simulink model "omav_LBF_bisection_combined"  (R2020a)
settings: Solver=VariableStepAuto  StartTime=0.0  StopTime=20  RelTol=1e-3
undefined symbols (not defined in the file): params
libraries: simulink x13, vrlib x2
settings Model: Creator=daniel  LastModifiedBy=daniel

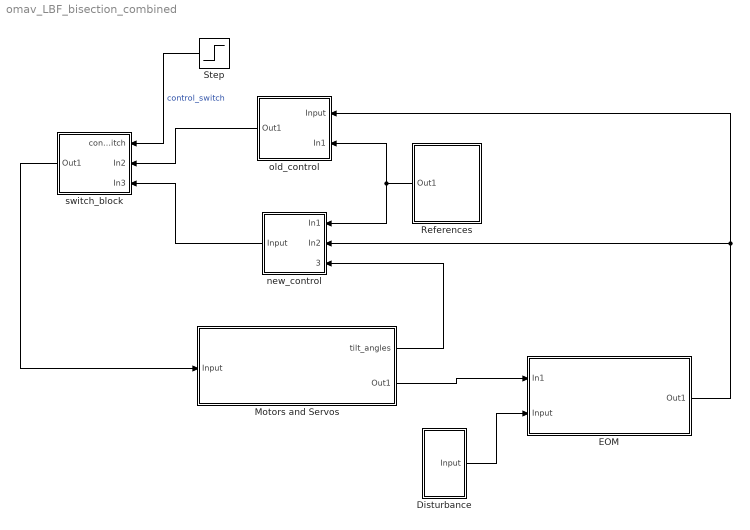
== system omav_LBF_bisection_combined ==
  Disturbance : Subsystem
  EOM : Subsystem
  Motors and Servos : Subsystem
  References : Subsystem
  Step : Step  Time=5  Before=1  After=0  SampleTime=0
  new_control : Subsystem
  old_control : Subsystem
  switch_block : Subsystem
  wires:
  EOM/1(Out1) -> old_control/1(Input), new_control/2(In2)
  References/1(Out1) -> old_control/2(In1), new_control/1(In1)
  Motors and Servos/2(Out1) -> EOM/1(In1)
  Disturbance/1(Input) -> EOM/2(Input)
  Motors and Servos/1(tilt_angles) -> new_control/3(tilt_angles)
  Step/1 -> switch_block/1(control_switch)  "control_switch"
  old_control/1(Out1) -> switch_block/2(In2)
  new_control/1(Input) -> switch_block/3(In3)
  switch_block/1(Out1) -> Motors and Servos/1(Input)

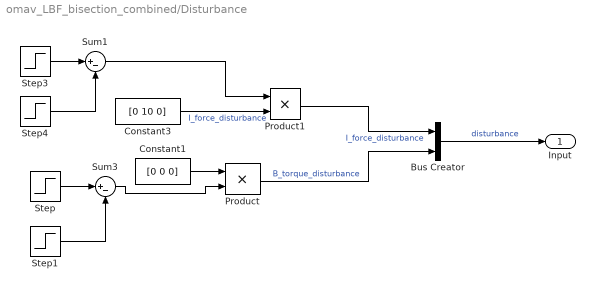
== system omav_LBF_bisection_combined/Disturbance ==
  Bus Creator : BusCreator  Inputs=2
  Constant1 : Constant  Value=[0 0 0]
  Constant3 : Constant  Value=[0 10 0]
  Product : Product
  Product1 : Product
  Step : Step  SampleTime=0
  Step1 : Step  Time=3  SampleTime=0
  Step3 : Step  Time=7  SampleTime=0
  Step4 : Step  Time=8  SampleTime=0
  Sum1 : Sum  Inputs=|+-
  Sum3 : Sum  Inputs=|+-
  Input : Outport
  wires:
  Product/1 -> Bus Creator/2  "B_torque_disturbance"
  Sum3/1 -> Product/2
  Constant1/1 -> Product/1
  Step/1 -> Sum3/1
  Product1/1 -> Bus Creator/1  "I_force_disturbance"
  Step1/1 -> Sum3/2
  Bus Creator/1 -> Input/1  "disturbance"
  Constant3/1 -> Product1/2  "I_force_disturbance"
  Sum1/1 -> Product1/1
  Step3/1 -> Sum1/1
  Step4/1 -> Sum1/2

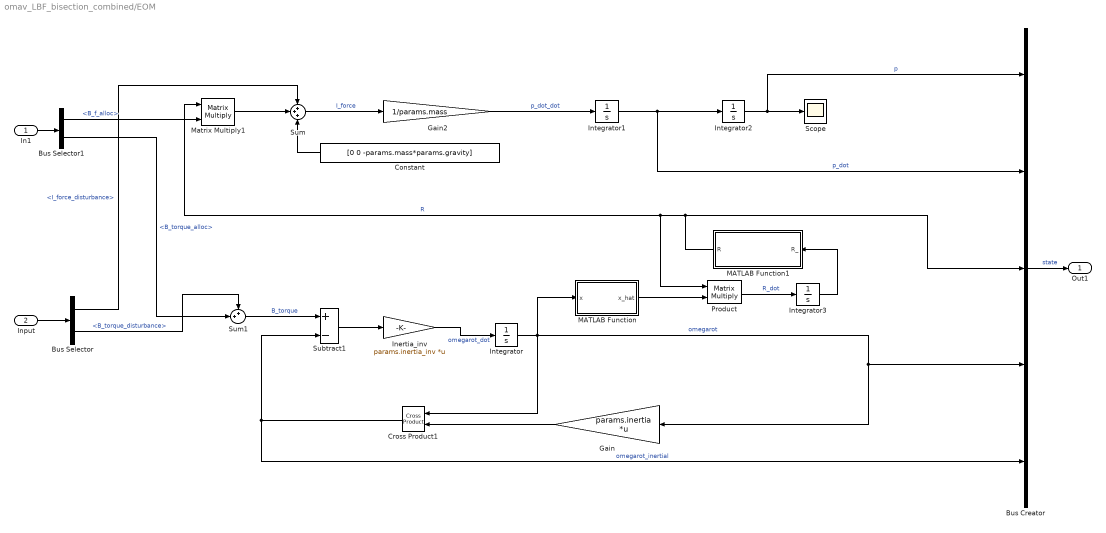
== system omav_LBF_bisection_combined/EOM ==
  In1 : Inport
  Input : Inport  Port=2
  Bus Creator : BusCreator  Inputs=5
  Bus Selector : BusSelector  OutputSignals=I_force_disturbance,B_torque_disturbance
  Bus Selector1 : BusSelector  OutputSignals=B_f_alloc,B_torque_alloc
  Constant : Constant  Value=[0 0 -params.mass*params.gravity]
  Cross Product1 : vrlib/Utilities/Cross Product
  Gain : Gain  Gain=params.inertia  Multiplication=Matrix(K*u) (u vector)
  Gain2 : Gain  Gain=1/params.mass
  Inertia_inv : Gain  Gain=params.inertia_inv  Multiplication=Matrix(K*u) (u vector)
  Integrator : Integrator
  Integrator1 : Integrator
  Integrator2 : Integrator
  Integrator3 : Integrator  InitialCondition=[1 0 0;0 1 0;0 0 1]
  MATLAB Function : MATLAB Function  TreatAsAtomicUnit=on
  MATLAB Function1 : MATLAB Function  TreatAsAtomicUnit=on
  Matrix Multiply1 : Product  Multiplication=Matrix(*)
  Product : Product  Multiplication=Matrix(*)  OutMin=0
  Scope : Scope
  Subtract1 : Sum  Inputs=+-
  Sum : Sum  Inputs=+++
  Sum1 : Sum  Inputs=++|
  Out1 : Outport
  wires:
  MATLAB Function/1(x_hat) -> Product/2
  Inertia_inv/1 -> Integrator/1  "omegarot_dot"
  Matrix Multiply1/1 -> Sum/2
  Sum1/1 -> Subtract1/1  "B_torque"
  Sum/1 -> Gain2/1  "I_force"
  Bus Selector/2 -> Sum1/1  "<B_torque_disturbance>"
  Constant/1 -> Sum/3
  MATLAB Function1/1(R) -> Product/1, Matrix Multiply1/1, Bus Creator/3  "R"
  Integrator2/1 -> Bus Creator/1, Scope/1  "p"
  Gain/1 -> Cross Product1/2
  Product/1 -> Integrator3/1  "R_dot"
  Subtract1/1 -> Inertia_inv/1
  Gain2/1 -> Integrator1/1  "p_dot_dot"
  Bus Selector1/1 -> Matrix Multiply1/2  "<B_f_alloc>"
  Cross Product1/1 -> Subtract1/2, Bus Creator/5  "omegarot_inertial"
  Bus Selector1/2 -> Sum1/2  "<B_torque_alloc>"
  Integrator/1 -> Gain/1, Bus Creator/4, MATLAB Function/1(x), Cross Product1/1  "omegarot"
  Bus Selector/1 -> Sum/1  "<I_force_disturbance>"
  Integrator1/1 -> Bus Creator/2, Integrator2/1  "p_dot"
  Integrator3/1 -> MATLAB Function1/1(R_)
  Bus Creator/1 -> Out1/1  "state"
  In1/1 -> Bus Selector1/1
  Input/1 -> Bus Selector/1

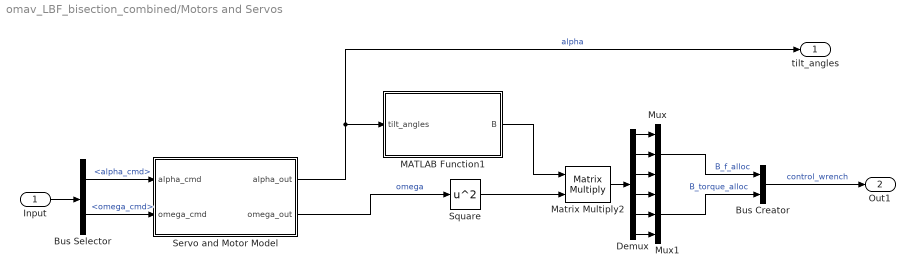
== system omav_LBF_bisection_combined/Motors and Servos ==
  Input : Inport
  Bus Creator : BusCreator  Inputs=2
  Bus Selector : BusSelector  OutputSignals=alpha_cmd,omega_cmd
  Demux : Demux  Outputs=6
  MATLAB Function1 : MATLAB Function  TreatAsAtomicUnit=on
  Matrix Multiply2 : Product  Multiplication=Matrix(*)
  Mux : Mux  Inputs=3
  Mux1 : Mux  Inputs=3
  Servo and Motor Model : Subsystem
  Square : Math  Operator=square  SaturateOnIntegerOverflow=on
  tilt_angles : Outport
  Out1 : Outport  Port=2
  wires:
  Demux/1 -> Mux/1
  MATLAB Function1/1(B) -> Matrix Multiply2/1
  Demux/4 -> Mux1/1
  Servo and Motor Model/2(omega_out) -> Square/1  "omega"
  Demux/5 -> Mux1/2
  Matrix Multiply2/1 -> Demux/1
  Servo and Motor Model/1(alpha_out) -> tilt_angles/1, MATLAB Function1/1(tilt_angles)  "alpha"
  Demux/6 -> Mux1/3
  Demux/2 -> Mux/2
  Square/1 -> Matrix Multiply2/2
  Mux/1 -> Bus Creator/1  "B_f_alloc"
  Demux/3 -> Mux/3
  Mux1/1 -> Bus Creator/2  "B_torque_alloc"
  Bus Creator/1 -> Out1/1  "control_wrench"
  Bus Selector/1 -> Servo and Motor Model/1(alpha_cmd)  "<alpha_cmd>"
  Bus Selector/2 -> Servo and Motor Model/2(omega_cmd)  "<omega_cmd>"
  Input/1 -> Bus Selector/1

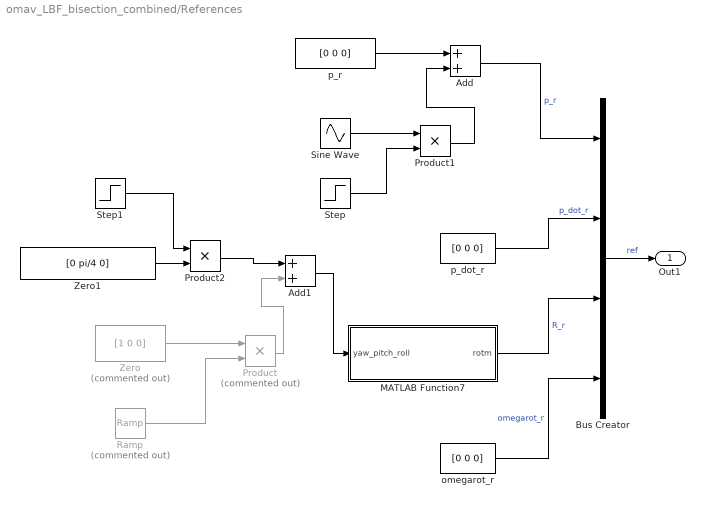
== system omav_LBF_bisection_combined/References ==
  Add : Sum
  Add1 : Sum
  Bus Creator : BusCreator  Inputs=4
  MATLAB Function7 : MATLAB Function  TreatAsAtomicUnit=on
  Product : Product  Commented=on
  Product1 : Product
  Product2 : Product
  Ramp : simulink/Sources/Ramp  Commented=on  slope=0.2  start=1  InitialOutput=0
  Sine Wave : Sin  Amplitude="[1 0  0]"  Phase=-3  SampleTime=0
  Step : Step  Time=3  SampleTime=0
  Step1 : Step  Time=0  SampleTime=0
  Zero : Constant  Commented=on  Value=[1 0 0]  OutDataTypeStr=Inherit: Inherit via back propagation
  Zero1 : Constant  Value=[0 pi/4 0]  OutDataTypeStr=Inherit: Inherit via back propagation
  omegarot_r : Constant  Value=[0 0 0]
  p_dot_r : Constant  Value=[0 0 0]
  p_r : Constant  Value=[0 0 0]
  Out1 : Outport
  wires:
  Step/1 -> Product1/2
  omegarot_r/1 -> Bus Creator/4  "omegarot_r"
  Add/1 -> Bus Creator/1  "p_r"
  MATLAB Function7/1(rotm) -> Bus Creator/3  "R_r"
  Product1/1 -> Add/2
  p_dot_r/1 -> Bus Creator/2  "p_dot_r"
  Sine Wave/1 -> Product1/1
  p_r/1 -> Add/1
  Zero/1 -> Product/1
  Bus Creator/1 -> Out1/1  "ref"
  Product/1 -> Add1/2
  Ramp/1 -> Product/2
  Add1/1 -> MATLAB Function7/1(yaw_pitch_roll)
  Zero1/1 -> Product2/2
  Product2/1 -> Add1/1
  Step1/1 -> Product2/1

== system omav_LBF_bisection_combined/new_control ==
  In1 : Inport
  In2 : Inport  Port=2
  tilt_angles : Inport  Port=3
  Attitude Control : Subsystem
  B_wrench_mapper : Subsystem
  Bus Creator1 : BusCreator  Inputs=2
  Mux : Mux  Inputs=2
  Position Control : Subsystem
  Input : Outport
  wires:
  Bus Creator1/1 -> Input/1  "commands"
  B_wrench_mapper/1(omega_cmd) -> Bus Creator1/2  "omega_cmd"
  Mux/1 -> B_wrench_mapper/2(wrench_b)
  In2/1 -> Position Control/2(In2), Attitude Control/2(Input)
  tilt_angles/1 -> Bus Creator1/1, Position Control/3(alpha_cmd), B_wrench_mapper/1(tilt_angles)
  In1/1 -> Position Control/1(In1), Attitude Control/1(In1)
  Attitude Control/1(B_torque_d) -> Mux/2
  Position Control/1(R_d) -> Attitude Control/3(Input1)
  Position Control/2(B_f_c) -> Mux/1  "B_f_c"

== system omav_LBF_bisection_combined/old_control ==
  Input : Inport
  In1 : Inport  Port=2
  A_allocation : Subsystem
  A_allocation_wrench : Subsystem
  Out1 : Outport
  wires:
  A_allocation/1(Out1) -> Out1/1
  Input/1 -> A_allocation_wrench/2(Input)
  A_allocation_wrench/1(A_wrench) -> A_allocation/1(wrench_b)
  In1/1 -> A_allocation_wrench/1(In1)

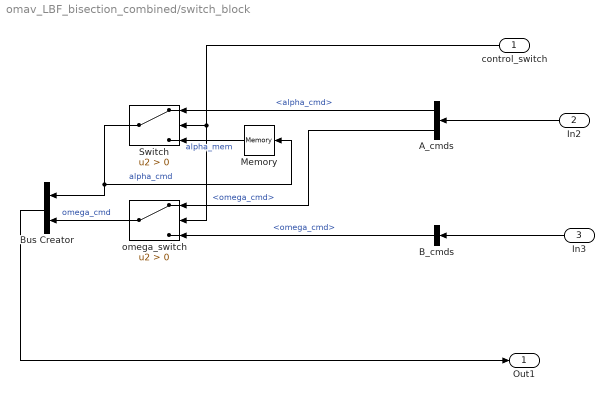
== system omav_LBF_bisection_combined/switch_block ==
  control_switch : Inport
  In2 : Inport  Port=2
  In3 : Inport  Port=3
  A_cmds : BusSelector  OutputSignals=alpha_cmd,omega_cmd
  B_cmds : BusSelector  OutputSignals=omega_cmd
  Bus Creator : BusCreator  Inputs=2
  Memory : Memory
  Switch : Switch  Criteria=u2 > Threshold
  omega_switch : Switch  Criteria=u2 > Threshold
  Out1 : Outport
  wires:
  B_cmds/1 -> omega_switch/3  "<omega_cmd>"
  A_cmds/2 -> omega_switch/1  "<omega_cmd>"
  Switch/1 -> Memory/1, Bus Creator/1  "alpha_cmd"
  omega_switch/1 -> Bus Creator/2  "omega_cmd"
  Memory/1 -> Switch/3  "alpha_mem"
  In2/1 -> A_cmds/1
  A_cmds/1 -> Switch/1  "<alpha_cmd>"
  Bus Creator/1 -> Out1/1
  In3/1 -> B_cmds/1
  control_switch/1 -> omega_switch/2, Switch/2

== system omav_LBF_bisection_combined/Motors and Servos/Servo and Motor Model ==
  alpha_cmd : Inport
  omega_cmd : Inport  Port=2
  all_rotors_subsystem1 : Subsystem
      mask Display: image('images/brushless.JPG'); % Use "Edit Image" on toolstrip to change.
  all_servos_subsystem1 : Subsystem
      mask Display: image('images/servo.jpg'); % Use "Edit Image" on toolstrip to change.
  alpha_out : Outport
  omega_out : Outport  Port=2
  wires:
  alpha_cmd/1 -> all_servos_subsystem1/1(alphas_cmd)  "alpha_cmd"
  all_rotors_subsystem1/1(omegas_out) -> omega_out/1  "omega_out"
  all_servos_subsystem1/1(alphas_out) -> alpha_out/1  "alpha_out"
  omega_cmd/1 -> all_rotors_subsystem1/1(omegas_cmd)  "omega_cmd"

== system omav_LBF_bisection_combined/new_control/Attitude Control ==
  In1 : Inport
  Input : Inport  Port=2
  Input1 : Inport  Port=3
  Bus Selector4 : BusSelector  OutputSignals=omegarot_r
  attitude_error_calculation : Subsystem
  B_torque_d : Outport
  wires:
  Input/1 -> attitude_error_calculation/1(Input)
  Bus Selector4/1 -> attitude_error_calculation/3(Input2)  "<omegarot_r>"
  In1/1 -> Bus Selector4/1
  Input1/1 -> attitude_error_calculation/2(Input1)
  attitude_error_calculation/1(B_torque_r) -> B_torque_d/1

== system omav_LBF_bisection_combined/new_control/B_wrench_mapper ==
  tilt_angles : Inport
  wrench_b : Inport  Port=2
  MATLAB Function2 : MATLAB Function  TreatAsAtomicUnit=on
  MATLAB Function6 : MATLAB Function  TreatAsAtomicUnit=on
  Sqrt : Sqrt  SaturateOnIntegerOverflow=on
  omega_cmd : Outport
  wires:
  wrench_b/1 -> MATLAB Function2/2(wrench_b)
  Sqrt/1 -> omega_cmd/1  "omega_cmd"
  MATLAB Function2/1(omega_sq) -> Sqrt/1
  MATLAB Function6/1(B) -> MATLAB Function2/1(B)
  tilt_angles/1 -> MATLAB Function6/1(tilt_angles)

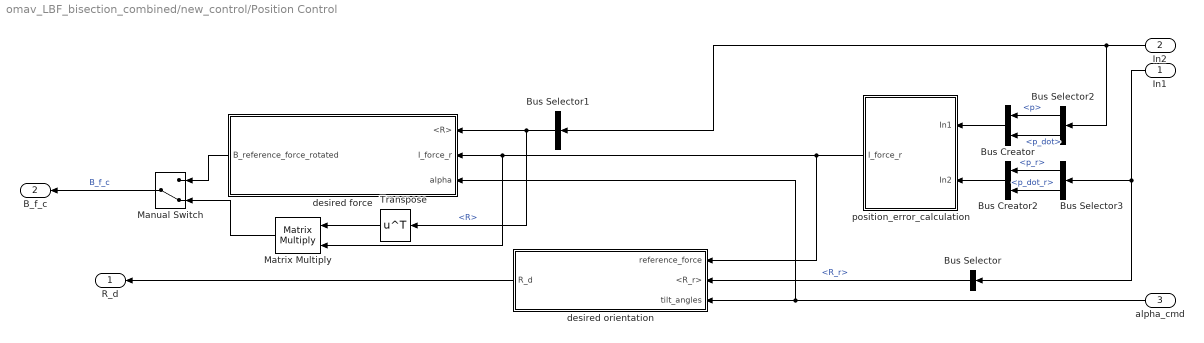
== system omav_LBF_bisection_combined/new_control/Position Control ==
  In1 : Inport
  In2 : Inport  Port=2
  alpha_cmd : Inport  Port=3
  Bus Creator2 : BusCreator  Inputs=2
  Bus Selector : BusSelector  OutputSignals=R_r
  Bus Selector1 : BusSelector  OutputSignals=R
  Bus Selector2 : BusSelector  OutputSignals=p,p_dot
  Bus Selector3 : BusSelector  OutputSignals=p_r,p_dot_r
  Bus Creator : BusCreator  Inputs=2
  Manual Switch : ManualSwitch  CurrentSetting=0
  Matrix Multiply : Product  Multiplication=Matrix(*)
  Transpose : Math  Operator=transpose  SaturateOnIntegerOverflow=on
  desired force : Subsystem
  desired orientation : Subsystem
  position_error_calculation : Subsystem
  R_d : Outport
  B_f_c : Outport  Port=2
  wires:
  Bus Selector3/1 -> Bus Creator2/1  "<p_r>"
  Bus Selector1/1 -> Transpose/1, desired force/1(<R>)  "<R>"
  desired orientation/1(R_d) -> R_d/1
  Bus Creator2/1 -> position_error_calculation/2(In2)
  In1/1 -> Bus Selector/1, Bus Selector3/1
  Manual Switch/1 -> B_f_c/1  "B_f_c"
  alpha_cmd/1 -> desired force/3(alpha), desired orientation/3(tilt_angles)
  Bus Selector/1 -> desired orientation/2(<R_r>)  "<R_r>"
  Bus Selector2/1 -> Bus Creator/1  "<p>"
  Bus Creator/1 -> position_error_calculation/1(In1)
  In2/1 -> Bus Selector2/1, Bus Selector1/1
  position_error_calculation/1(I_force_r) -> desired orientation/1(reference_force), Matrix Multiply/2, desired force/2(I_force_r)
  Bus Selector3/2 -> Bus Creator2/2  "<p_dot_r>"
  Bus Selector2/2 -> Bus Creator/2  "<p_dot>"
  desired force/1(B_reference_force_rotated) -> Manual Switch/1
  Matrix Multiply/1 -> Manual Switch/2
  Transpose/1 -> Matrix Multiply/1

== system omav_LBF_bisection_combined/old_control/A_allocation ==
  wrench_b : Inport
  Bus Creator : BusCreator  Inputs=2
  MATLAB Function3 : MATLAB Function  TreatAsAtomicUnit=on
  MATLAB Function4 : MATLAB Function  TreatAsAtomicUnit=on
  MATLAB Function5 : MATLAB Function  TreatAsAtomicUnit=on
  Sqrt : Sqrt  SaturateOnIntegerOverflow=on
  Out1 : Outport
  wires:
  MATLAB Function5/1(X) -> MATLAB Function4/1(X)
  wrench_b/1 -> MATLAB Function5/2(wrench_b)
  MATLAB Function4/2(omegas_sq) -> Sqrt/1
  MATLAB Function4/1(alphas) -> Bus Creator/1  "alpha_cmd"
  MATLAB Function3/1(A) -> MATLAB Function5/1(A)
  Bus Creator/1 -> Out1/1  "commands"
  Sqrt/1 -> Bus Creator/2  "omega_cmd"

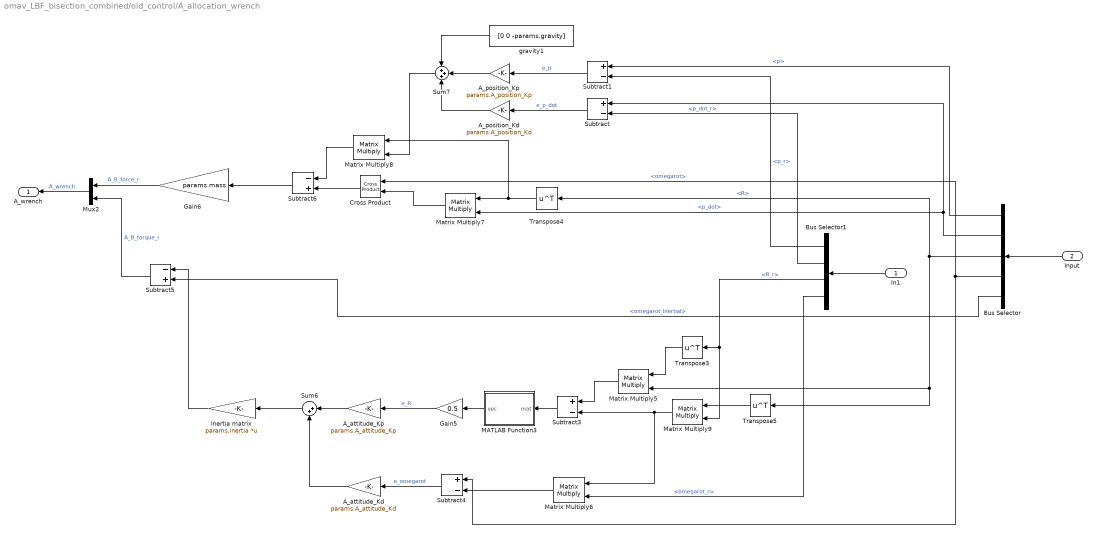
== system omav_LBF_bisection_combined/old_control/A_allocation_wrench ==
  In1 : Inport
  Input : Inport  Port=2
  A_attitude_Kd : Gain  Gain=params.A_attitude_Kd
  A_attitude_Kp : Gain  Gain=params.A_attitude_Kp
  A_position_Kd : Gain  Gain=params.A_position_Kd
  A_position_Kp : Gain  Gain=params.A_position_Kp
  Bus Selector : BusSelector  OutputSignals=p,p_dot,R,omegarot,omegarot_inertial
  Bus Selector1 : BusSelector  OutputSignals=p_r,p_dot_r,R_r,omegarot_r
  Cross Product : vrlib/Utilities/Cross Product
  Gain5 : Gain  Gain=0.5
  Gain6 : Gain  Gain=params.mass
  Inertia matrix : Gain  Gain=params.inertia  Multiplication=Matrix(K*u) (u vector)
  MATLAB Function3 : MATLAB Function  TreatAsAtomicUnit=on
  Matrix Multiply{5..9} (5 alike) : Product  Multiplication=Matrix(*)
  Mux2 : Mux  Inputs=2
  Subtract{,1,3..4} (4 alike) : Sum  Inputs=+-
  Subtract5 : Sum  Inputs=-+
  Subtract6 : Sum  Inputs=-+
  Sum6 : Sum  Inputs=|++
  Sum7 : Sum  Inputs=+++
  Transpose3 : Math  Operator=transpose  SaturateOnIntegerOverflow=on
  Transpose4 : Math  Operator=transpose  SaturateOnIntegerOverflow=on
  Transpose5 : Math  Operator=transpose  SaturateOnIntegerOverflow=on
  gravity1 : Constant  Value=[0 0 -params.gravity]
  A_wrench : Outport
  wires:
  A_position_Kd/1 -> Sum7/3
  Bus Selector1/2 -> Subtract/2  "<p_dot_r>"
  Subtract5/1 -> Mux2/2  "A_B_torque_r"
  Inertia matrix/1 -> Subtract5/1
  Subtract4/1 -> A_attitude_Kd/1  "e_omegarot"
  gravity1/1 -> Sum7/1
  Transpose3/1 -> Matrix Multiply5/1
  Subtract6/1 -> Gain6/1
  Cross Product/1 -> Subtract6/2
  Subtract3/1 -> MATLAB Function3/1(mat)
  Bus Selector1/3 -> Matrix Multiply9/2, Transpose3/1  "<R_r>"
  Subtract1/1 -> A_position_Kp/1  "e_p"
  A_attitude_Kd/1 -> Sum6/2
  Input/1 -> Bus Selector/1
  A_position_Kp/1 -> Sum7/2
  Transpose4/1 -> Matrix Multiply8/1, Matrix Multiply7/1
  Matrix Multiply8/1 -> Subtract6/1
  Gain5/1 -> A_attitude_Kp/1  "e_R"
  Mux2/1 -> A_wrench/1  "A_wrench"
  A_attitude_Kp/1 -> Sum6/1
  MATLAB Function3/1(vec) -> Gain5/1
  In1/1 -> Bus Selector1/1
  Matrix Multiply5/1 -> Subtract3/1
  Gain6/1 -> Mux2/1  "A_B_force_r"
  Bus Selector1/4 -> Matrix Multiply6/2  "<omegarot_r>"
  Sum6/1 -> Inertia matrix/1
  Matrix Multiply6/1 -> Subtract4/2
  Sum7/1 -> Matrix Multiply8/2
  Matrix Multiply9/1 -> Subtract3/2, Matrix Multiply6/1
  Matrix Multiply7/1 -> Cross Product/2
  Transpose5/1 -> Matrix Multiply9/1
  Bus Selector1/1 -> Subtract1/2  "<p_r>"
  Subtract/1 -> A_position_Kd/1  "e_p_dot"
  Bus Selector/1 -> Subtract1/1  "<p>"
  Bus Selector/2 -> Subtract/1, Matrix Multiply7/2  "<p_dot>"
  Bus Selector/3 -> Matrix Multiply5/2, Transpose5/1, Transpose4/1  "<R>"
  Bus Selector/4 -> Subtract4/1, Cross Product/1  "<omegarot>"
  Bus Selector/5 -> Subtract5/2  "<omegarot_inertial>"

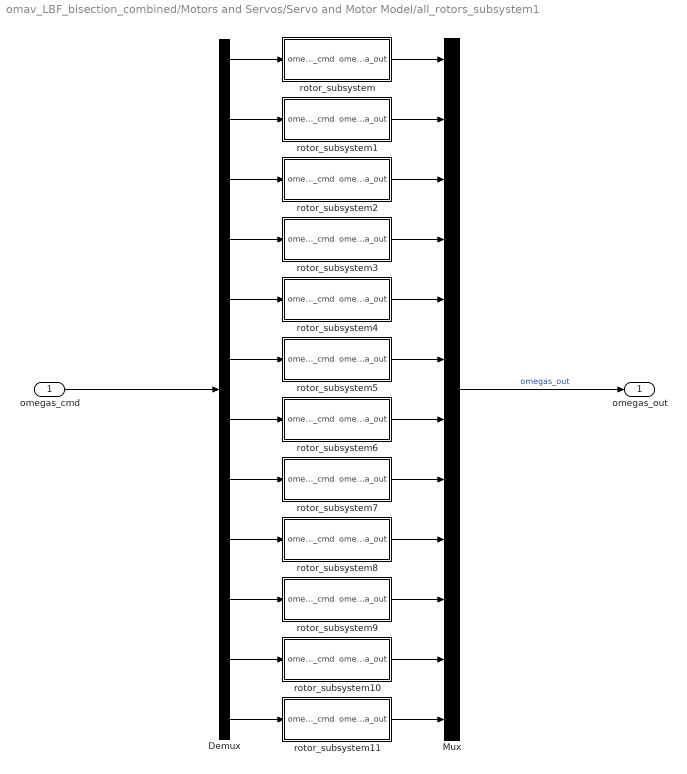
== system omav_LBF_bisection_combined/Motors and Servos/Servo and Motor Model/all_rotors_subsystem1 ==
  omegas_cmd : Inport
  Demux : Demux  Outputs=12
  Mux : Mux  Inputs=12
  rotor_subsystem : Subsystem
  rotor_subsystem1 : Subsystem
  rotor_subsystem10 : Subsystem
  rotor_subsystem11 : Subsystem
  rotor_subsystem2 : Subsystem
  rotor_subsystem3 : Subsystem
  rotor_subsystem4 : Subsystem
  rotor_subsystem5 : Subsystem
  rotor_subsystem6 : Subsystem
  rotor_subsystem7 : Subsystem
  rotor_subsystem8 : Subsystem
  rotor_subsystem9 : Subsystem
  omegas_out : Outport
  wires:
  Demux/3 -> rotor_subsystem2/1(omega_cmd)
  rotor_subsystem10/1(omega_out) -> Mux/11
  rotor_subsystem7/1(omega_out) -> Mux/8
  rotor_subsystem2/1(omega_out) -> Mux/3
  rotor_subsystem1/1(omega_out) -> Mux/2
  Demux/2 -> rotor_subsystem1/1(omega_cmd)
  rotor_subsystem5/1(omega_out) -> Mux/6
  rotor_subsystem4/1(omega_out) -> Mux/5
  Demux/4 -> rotor_subsystem3/1(omega_cmd)
  rotor_subsystem6/1(omega_out) -> Mux/7
  Demux/8 -> rotor_subsystem7/1(omega_cmd)
  rotor_subsystem/1(omega_out) -> Mux/1
  rotor_subsystem3/1(omega_out) -> Mux/4
  rotor_subsystem11/1(omega_out) -> Mux/12
  rotor_subsystem8/1(omega_out) -> Mux/9
  Demux/11 -> rotor_subsystem10/1(omega_cmd)
  rotor_subsystem9/1(omega_out) -> Mux/10
  Demux/1 -> rotor_subsystem/1(omega_cmd)
  omegas_cmd/1 -> Demux/1
  Mux/1 -> omegas_out/1  "omegas_out"
  Demux/12 -> rotor_subsystem11/1(omega_cmd)
  Demux/10 -> rotor_subsystem9/1(omega_cmd)
  Demux/9 -> rotor_subsystem8/1(omega_cmd)
  Demux/7 -> rotor_subsystem6/1(omega_cmd)
  Demux/6 -> rotor_subsystem5/1(omega_cmd)
  Demux/5 -> rotor_subsystem4/1(omega_cmd)

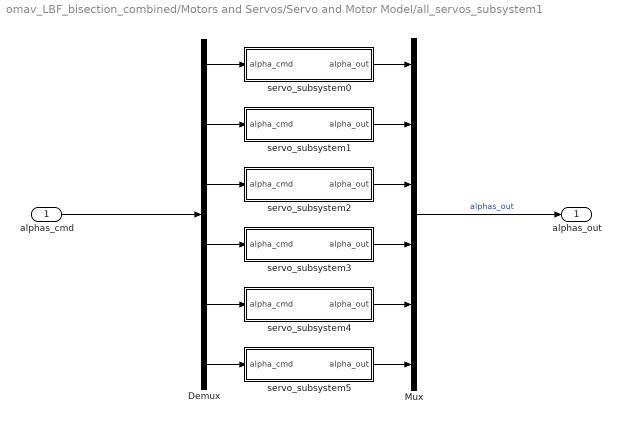
== system omav_LBF_bisection_combined/Motors and Servos/Servo and Motor Model/all_servos_subsystem1 ==
  alphas_cmd : Inport
  Demux : Demux  Outputs=6
  Mux : Mux  Inputs=6
  servo_subsystem0 : Subsystem
  servo_subsystem1 : Subsystem
  servo_subsystem2 : Subsystem
  servo_subsystem3 : Subsystem
  servo_subsystem4 : Subsystem
  servo_subsystem5 : Subsystem
  alphas_out : Outport
  wires:
  alphas_cmd/1 -> Demux/1
  Demux/2 -> servo_subsystem1/1(alpha_cmd)
  servo_subsystem3/1(alpha_out) -> Mux/4
  servo_subsystem1/1(alpha_out) -> Mux/2
  Demux/4 -> servo_subsystem3/1(alpha_cmd)
  servo_subsystem4/1(alpha_out) -> Mux/5
  Demux/5 -> servo_subsystem4/1(alpha_cmd)
  Demux/1 -> servo_subsystem0/1(alpha_cmd)
  servo_subsystem2/1(alpha_out) -> Mux/3
  servo_subsystem5/1(alpha_out) -> Mux/6
  Demux/6 -> servo_subsystem5/1(alpha_cmd)
  Demux/3 -> servo_subsystem2/1(alpha_cmd)
  Mux/1 -> alphas_out/1  "alphas_out"
  servo_subsystem0/1(alpha_out) -> Mux/1

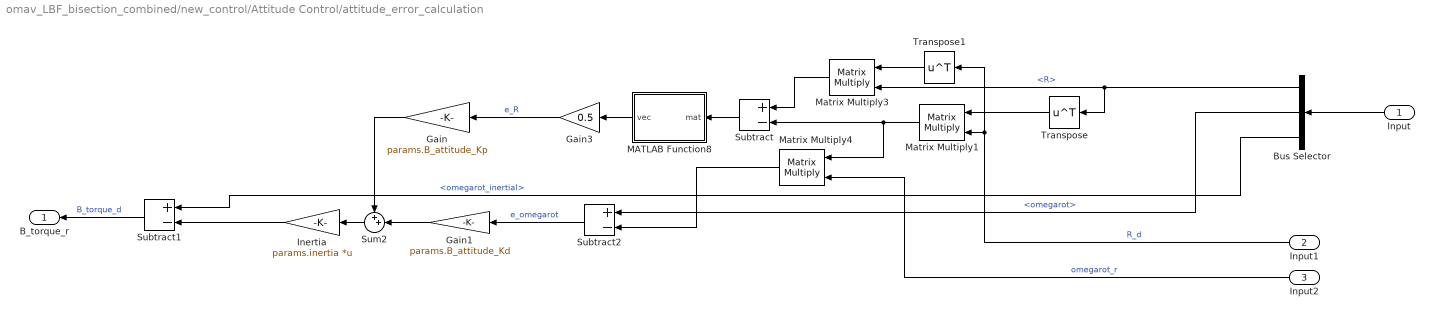
== system omav_LBF_bisection_combined/new_control/Attitude Control/attitude_error_calculation ==
  Input : Inport
  Input1 : Inport  Port=2
  Input2 : Inport  Port=3
  Bus Selector : BusSelector  OutputSignals=R,omegarot,omegarot_inertial
  Gain : Gain  Gain=params.B_attitude_Kp
  Gain1 : Gain  Gain=params.B_attitude_Kd
  Gain3 : Gain  Gain=0.5
  Inertia : Gain  Gain=params.inertia  Multiplication=Matrix(K*u) (u vector)
  MATLAB Function8 : MATLAB Function  TreatAsAtomicUnit=on
  Matrix Multiply1 : Product  Multiplication=Matrix(*)
  Matrix Multiply3 : Product  Multiplication=Matrix(*)
  Matrix Multiply4 : Product  Multiplication=Matrix(*)
  Subtract : Sum  Inputs=+-
  Subtract1 : Sum  Inputs=+-
  Subtract2 : Sum  Inputs=+-
  Sum2 : Sum  Inputs=++|
  Transpose : Math  Operator=transpose  SaturateOnIntegerOverflow=on
  Transpose1 : Math  Operator=transpose  SaturateOnIntegerOverflow=on
  B_torque_r : Outport
  wires:
  Subtract1/1 -> B_torque_r/1  "B_torque_d"
  Transpose1/1 -> Matrix Multiply3/1
  Gain/1 -> Sum2/1
  Matrix Multiply4/1 -> Subtract2/2
  Transpose/1 -> Matrix Multiply1/1
  Input2/1 -> Matrix Multiply4/2  "omegarot_r"
  Bus Selector/3 -> Subtract1/1  "<omegarot_inertial>"
  MATLAB Function8/1(vec) -> Gain3/1
  Input1/1 -> Matrix Multiply1/2, Transpose1/1  "R_d"
  Bus Selector/1 -> Transpose/1, Matrix Multiply3/2  "<R>"
  Subtract/1 -> MATLAB Function8/1(mat)
  Matrix Multiply3/1 -> Subtract/1
  Inertia/1 -> Subtract1/2
  Gain3/1 -> Gain/1  "e_R"
  Matrix Multiply1/1 -> Subtract/2, Matrix Multiply4/1
  Subtract2/1 -> Gain1/1  "e_omegarot"
  Gain1/1 -> Sum2/2
  Bus Selector/2 -> Subtract2/1  "<omegarot>"
  Sum2/1 -> Inertia/1
  Input/1 -> Bus Selector/1

== system omav_LBF_bisection_combined/new_control/Position Control/desired force ==
  <R> : Inport
  I_force_r : Inport  Port=2
  alpha : Inport  Port=3
  MATLAB Function : MATLAB Function  TreatAsAtomicUnit=on
  MATLAB Function1 : MATLAB Function  TreatAsAtomicUnit=on
  Scope : Scope
  B_reference_force_rotated : Outport
  wires:
  MATLAB Function/1(B_f_c) -> B_reference_force_rotated/1
  I_force_r/1 -> MATLAB Function/2(I_f_r)
  <R>/1 -> MATLAB Function/3(R)
  MATLAB Function1/1(B) -> MATLAB Function/1(B)
  alpha/1 -> MATLAB Function1/1(tilt_angles)
  MATLAB Function/2(lambda) -> Scope/1  "lambda_f"

== system omav_LBF_bisection_combined/new_control/Position Control/desired orientation ==
  reference_force : Inport
  <R_r> : Inport  Port=2
  tilt_angles : Inport  Port=3
  MATLAB Function1 : MATLAB Function  TreatAsAtomicUnit=on
  MATLAB Function2 : MATLAB Function  TreatAsAtomicUnit=on
  Matrix Multiply2 : Product  Multiplication=Matrix(*)
  Scope : Scope
  R_d : Outport
  wires:
  reference_force/1 -> MATLAB Function1/3(I_f_r)
  Matrix Multiply2/1 -> R_d/1  "R_d"
  MATLAB Function1/1(R_s) -> Matrix Multiply2/2  "B_search_rotmat"
  <R_r>/1 -> Matrix Multiply2/1, MATLAB Function1/2(R_r)
  tilt_angles/1 -> MATLAB Function2/1(tilt_angles)
  MATLAB Function2/1(B) -> MATLAB Function1/1(B)
  MATLAB Function1/2(lambda) -> Scope/1  "lambda_R"

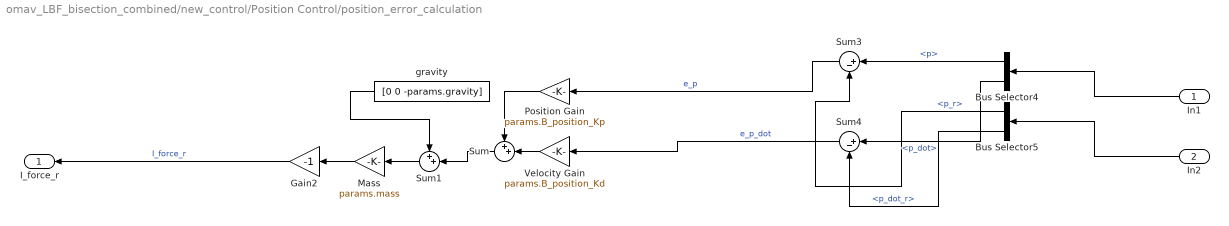
== system omav_LBF_bisection_combined/new_control/Position Control/position_error_calculation ==
  In1 : Inport
  In2 : Inport  Port=2
  Bus Selector4 : BusSelector  OutputSignals=p,p_dot
  Bus Selector5 : BusSelector  OutputSignals=p_r,p_dot_r
  Gain2 : Gain  Gain=-1
  Mass : Gain  Gain=params.mass
  Position Gain : Gain  Gain=params.B_position_Kp
  Sum : Sum  Inputs=++|
  Sum1 : Sum  Inputs=++|
  Sum3 : Sum  Inputs=|+-
  Sum4 : Sum  Inputs=|+-
  Velocity Gain : Gain  Gain=params.B_position_Kd
  gravity : Constant  Value=[0 0 -params.gravity]
  I_force_r : Outport
  wires:
  Sum1/1 -> Mass/1
  gravity/1 -> Sum1/1
  Bus Selector4/2 -> Sum4/1  "<p_dot>"
  Velocity Gain/1 -> Sum/2
  Bus Selector5/2 -> Sum4/2  "<p_dot_r>"
  Gain2/1 -> I_force_r/1  "I_force_r"
  Sum/1 -> Sum1/2
  In1/1 -> Bus Selector4/1
  Mass/1 -> Gain2/1
  Sum4/1 -> Velocity Gain/1  "e_p_dot"
  Position Gain/1 -> Sum/1
  In2/1 -> Bus Selector5/1
  Sum3/1 -> Position Gain/1  "e_p"
  Bus Selector4/1 -> Sum3/1  "<p>"
  Bus Selector5/1 -> Sum3/2  "<p_r>"

== system omav_LBF_bisection_combined/Motors and Servos/Servo and Motor Model/all_rotors_subsystem1/rotor_subsystem ==
  omega_cmd : Inport
  Detect Increase : simulink/Logic and Bit Operations/Detect Increase  vinit=0.0  OutDataTypeStr=boolean
  Saturation : Saturate  UpperLimit=params.rotor_max  LowerLimit=0
  Switch : Switch  Criteria=u2 > Threshold
  down : TransferFcn  Numerator=[88]  Denominator=[1 88]
  up : TransferFcn  Numerator=[176]  Denominator=[1 176]
  omega_out : Outport
  wires:
  down/1 -> Switch/3
  up/1 -> Detect Increase/1, Switch/1
  omega_cmd/1 -> up/1, down/1
  Switch/1 -> Saturation/1
  Detect Increase/1 -> Switch/2
  Saturation/1 -> omega_out/1  "omega_out"

== system omav_LBF_bisection_combined/Motors and Servos/Servo and Motor Model/all_rotors_subsystem1/rotor_subsystem1 ==
  omega_cmd : Inport
  Detect Increase : simulink/Logic and Bit Operations/Detect Increase  vinit=0.0  OutDataTypeStr=boolean
  Saturation : Saturate  UpperLimit=params.rotor_max  LowerLimit=0
  Switch : Switch  Criteria=u2 > Threshold
  down : TransferFcn  Numerator=[88]  Denominator=[1 88]
  up : TransferFcn  Numerator=[176]  Denominator=[1 176]
  omega_out : Outport
  wires:
  Saturation/1 -> omega_out/1  "omega_out"
  Detect Increase/1 -> Switch/2
  Switch/1 -> Saturation/1
  omega_cmd/1 -> down/1, up/1
  up/1 -> Switch/1, Detect Increase/1
  down/1 -> Switch/3

== system omav_LBF_bisection_combined/Motors and Servos/Servo and Motor Model/all_rotors_subsystem1/rotor_subsystem10 ==
  omega_cmd : Inport
  Detect Increase : simulink/Logic and Bit Operations/Detect Increase  vinit=0.0  OutDataTypeStr=boolean
  Saturation : Saturate  UpperLimit=params.rotor_max  LowerLimit=0
  Switch : Switch  Criteria=u2 > Threshold
  down : TransferFcn  Numerator=[88]  Denominator=[1 88]
  up : TransferFcn  Numerator=[176]  Denominator=[1 176]
  omega_out : Outport
  wires:
  down/1 -> Switch/3
  up/1 -> Detect Increase/1, Switch/1
  omega_cmd/1 -> up/1, down/1
  Switch/1 -> Saturation/1
  Detect Increase/1 -> Switch/2
  Saturation/1 -> omega_out/1  "omega_out"

== system omav_LBF_bisection_combined/Motors and Servos/Servo and Motor Model/all_rotors_subsystem1/rotor_subsystem11 ==
  omega_cmd : Inport
  Detect Increase : simulink/Logic and Bit Operations/Detect Increase  vinit=0.0  OutDataTypeStr=boolean
  Saturation : Saturate  UpperLimit=params.rotor_max  LowerLimit=0
  Switch : Switch  Criteria=u2 > Threshold
  down : TransferFcn  Numerator=[88]  Denominator=[1 88]
  up : TransferFcn  Numerator=[176]  Denominator=[1 176]
  omega_out : Outport
  wires:
  Saturation/1 -> omega_out/1  "omega_out"
  Detect Increase/1 -> Switch/2
  Switch/1 -> Saturation/1
  omega_cmd/1 -> down/1, up/1
  up/1 -> Switch/1, Detect Increase/1
  down/1 -> Switch/3

== system omav_LBF_bisection_combined/Motors and Servos/Servo and Motor Model/all_rotors_subsystem1/rotor_subsystem2 ==
  omega_cmd : Inport
  Detect Increase : simulink/Logic and Bit Operations/Detect Increase  vinit=0.0  OutDataTypeStr=boolean
  Saturation : Saturate  UpperLimit=params.rotor_max  LowerLimit=0
  Switch : Switch  Criteria=u2 > Threshold
  down : TransferFcn  Numerator=[88]  Denominator=[1 88]
  up : TransferFcn  Numerator=[176]  Denominator=[1 176]
  omega_out : Outport
  wires:
  down/1 -> Switch/3
  up/1 -> Detect Increase/1, Switch/1
  omega_cmd/1 -> up/1, down/1
  Switch/1 -> Saturation/1
  Detect Increase/1 -> Switch/2
  Saturation/1 -> omega_out/1  "omega_out"

== system omav_LBF_bisection_combined/Motors and Servos/Servo and Motor Model/all_rotors_subsystem1/rotor_subsystem3 ==
  omega_cmd : Inport
  Detect Increase : simulink/Logic and Bit Operations/Detect Increase  vinit=0.0  OutDataTypeStr=boolean
  Saturation : Saturate  UpperLimit=params.rotor_max  LowerLimit=0
  Switch : Switch  Criteria=u2 > Threshold
  down : TransferFcn  Numerator=[88]  Denominator=[1 88]
  up : TransferFcn  Numerator=[176]  Denominator=[1 176]
  omega_out : Outport
  wires:
  Saturation/1 -> omega_out/1  "omega_out"
  Detect Increase/1 -> Switch/2
  Switch/1 -> Saturation/1
  omega_cmd/1 -> down/1, up/1
  up/1 -> Switch/1, Detect Increase/1
  down/1 -> Switch/3

== system omav_LBF_bisection_combined/Motors and Servos/Servo and Motor Model/all_rotors_subsystem1/rotor_subsystem4 ==
  omega_cmd : Inport
  Detect Increase : simulink/Logic and Bit Operations/Detect Increase  vinit=0.0  OutDataTypeStr=boolean
  Saturation : Saturate  UpperLimit=params.rotor_max  LowerLimit=0
  Switch : Switch  Criteria=u2 > Threshold
  down : TransferFcn  Numerator=[88]  Denominator=[1 88]
  up : TransferFcn  Numerator=[176]  Denominator=[1 176]
  omega_out : Outport
  wires:
  down/1 -> Switch/3
  up/1 -> Detect Increase/1, Switch/1
  omega_cmd/1 -> up/1, down/1
  Switch/1 -> Saturation/1
  Detect Increase/1 -> Switch/2
  Saturation/1 -> omega_out/1  "omega_out"

== system omav_LBF_bisection_combined/Motors and Servos/Servo and Motor Model/all_rotors_subsystem1/rotor_subsystem5 ==
  omega_cmd : Inport
  Detect Increase : simulink/Logic and Bit Operations/Detect Increase  vinit=0.0  OutDataTypeStr=boolean
  Saturation : Saturate  UpperLimit=params.rotor_max  LowerLimit=0
  Switch : Switch  Criteria=u2 > Threshold
  down : TransferFcn  Numerator=[88]  Denominator=[1 88]
  up : TransferFcn  Numerator=[176]  Denominator=[1 176]
  omega_out : Outport
  wires:
  Saturation/1 -> omega_out/1  "omega_out"
  Detect Increase/1 -> Switch/2
  Switch/1 -> Saturation/1
  omega_cmd/1 -> down/1, up/1
  up/1 -> Switch/1, Detect Increase/1
  down/1 -> Switch/3

== system omav_LBF_bisection_combined/Motors and Servos/Servo and Motor Model/all_rotors_subsystem1/rotor_subsystem6 ==
  omega_cmd : Inport
  Detect Increase : simulink/Logic and Bit Operations/Detect Increase  vinit=0.0  OutDataTypeStr=boolean
  Saturation : Saturate  UpperLimit=params.rotor_max  LowerLimit=0
  Switch : Switch  Criteria=u2 > Threshold
  down : TransferFcn  Numerator=[88]  Denominator=[1 88]
  up : TransferFcn  Numerator=[176]  Denominator=[1 176]
  omega_out : Outport
  wires:
  down/1 -> Switch/3
  up/1 -> Detect Increase/1, Switch/1
  omega_cmd/1 -> up/1, down/1
  Switch/1 -> Saturation/1
  Detect Increase/1 -> Switch/2
  Saturation/1 -> omega_out/1  "omega_out"

== system omav_LBF_bisection_combined/Motors and Servos/Servo and Motor Model/all_rotors_subsystem1/rotor_subsystem7 ==
  omega_cmd : Inport
  Detect Increase : simulink/Logic and Bit Operations/Detect Increase  vinit=0.0  OutDataTypeStr=boolean
  Saturation : Saturate  UpperLimit=params.rotor_max  LowerLimit=0
  Switch : Switch  Criteria=u2 > Threshold
  down : TransferFcn  Numerator=[88]  Denominator=[1 88]
  up : TransferFcn  Numerator=[176]  Denominator=[1 176]
  omega_out : Outport
  wires:
  Saturation/1 -> omega_out/1  "omega_out"
  Detect Increase/1 -> Switch/2
  Switch/1 -> Saturation/1
  omega_cmd/1 -> down/1, up/1
  up/1 -> Switch/1, Detect Increase/1
  down/1 -> Switch/3

== system omav_LBF_bisection_combined/Motors and Servos/Servo and Motor Model/all_rotors_subsystem1/rotor_subsystem8 ==
  omega_cmd : Inport
  Detect Increase : simulink/Logic and Bit Operations/Detect Increase  vinit=0.0  OutDataTypeStr=boolean
  Saturation : Saturate  UpperLimit=params.rotor_max  LowerLimit=0
  Switch : Switch  Criteria=u2 > Threshold
  down : TransferFcn  Numerator=[88]  Denominator=[1 88]
  up : TransferFcn  Numerator=[176]  Denominator=[1 176]
  omega_out : Outport
  wires:
  down/1 -> Switch/3
  up/1 -> Detect Increase/1, Switch/1
  omega_cmd/1 -> up/1, down/1
  Switch/1 -> Saturation/1
  Detect Increase/1 -> Switch/2
  Saturation/1 -> omega_out/1  "omega_out"

== system omav_LBF_bisection_combined/Motors and Servos/Servo and Motor Model/all_rotors_subsystem1/rotor_subsystem9 ==
  omega_cmd : Inport
  Detect Increase : simulink/Logic and Bit Operations/Detect Increase  vinit=0.0  OutDataTypeStr=boolean
  Saturation : Saturate  UpperLimit=params.rotor_max  LowerLimit=0
  Switch : Switch  Criteria=u2 > Threshold
  down : TransferFcn  Numerator=[88]  Denominator=[1 88]
  up : TransferFcn  Numerator=[176]  Denominator=[1 176]
  omega_out : Outport
  wires:
  Saturation/1 -> omega_out/1  "omega_out"
  Detect Increase/1 -> Switch/2
  Switch/1 -> Saturation/1
  omega_cmd/1 -> down/1, up/1
  up/1 -> Switch/1, Detect Increase/1
  down/1 -> Switch/3

== system omav_LBF_bisection_combined/Motors and Servos/Servo and Motor Model/all_servos_subsystem1/servo_subsystem0 ==
  alpha_cmd : Inport
  Servo Transfer Function : TransferFcn  Numerator=[256]  Denominator=[1 22.4 256]
  alpha_out : Outport
  wires:
  alpha_cmd/1 -> Servo Transfer Function/1
  Servo Transfer Function/1 -> alpha_out/1  "alpha_out"

== system omav_LBF_bisection_combined/Motors and Servos/Servo and Motor Model/all_servos_subsystem1/servo_subsystem1 ==
  alpha_cmd : Inport
  Servo Transfer Function : TransferFcn  Numerator=[256]  Denominator=[1 22.4 256]
  alpha_out : Outport
  wires:
  Servo Transfer Function/1 -> alpha_out/1  "alpha_out"
  alpha_cmd/1 -> Servo Transfer Function/1

== system omav_LBF_bisection_combined/Motors and Servos/Servo and Motor Model/all_servos_subsystem1/servo_subsystem2 ==
  alpha_cmd : Inport
  Servo Transfer Function : TransferFcn  Numerator=[256]  Denominator=[1 22.4 256]
  alpha_out : Outport
  wires:
  alpha_cmd/1 -> Servo Transfer Function/1
  Servo Transfer Function/1 -> alpha_out/1  "alpha_out"

== system omav_LBF_bisection_combined/Motors and Servos/Servo and Motor Model/all_servos_subsystem1/servo_subsystem3 ==
  alpha_cmd : Inport
  Servo Transfer Function : TransferFcn  Numerator=[256]  Denominator=[1 22.4 256]
  alpha_out : Outport
  wires:
  Servo Transfer Function/1 -> alpha_out/1  "alpha_out"
  alpha_cmd/1 -> Servo Transfer Function/1

== system omav_LBF_bisection_combined/Motors and Servos/Servo and Motor Model/all_servos_subsystem1/servo_subsystem4 ==
  alpha_cmd : Inport
  Servo Transfer Function : TransferFcn  Numerator=[256]  Denominator=[1 22.4 256]
  alpha_out : Outport
  wires:
  alpha_cmd/1 -> Servo Transfer Function/1
  Servo Transfer Function/1 -> alpha_out/1  "alpha_out"

== system omav_LBF_bisection_combined/Motors and Servos/Servo and Motor Model/all_servos_subsystem1/servo_subsystem5 ==
  alpha_cmd : Inport
  Servo Transfer Function : TransferFcn  Numerator=[256]  Denominator=[1 22.4 256]
  alpha_out : Outport
  wires:
  Servo Transfer Function/1 -> alpha_out/1  "alpha_out"
  alpha_cmd/1 -> Servo Transfer Function/1

== matlab function omav_LBF_bisection_combined/new_control/Position Control/desired orientation/MATLAB Function2 ==
  data: tilt_angles input; B output
function B = get_B(tilt_angles)
%tilt_angles [6x1]
%[F, tau] = B * [omega²]

params = parameters();

rotor_force_constant = params.rotor_force_constant;
rotor_moment_constant = params.rotor_moment_constant;
arm_length = params.arm_length;

arm_angles = params.arm_angles;
spin = params.spin;

B = zeros(6,12);


j = 0;

%repeat every tilt angle
rep_tilt_angles = repelem(tilt_angles,2);
%iterating through every rotor
%refactored to z-upwards
for i = 1:12
  
    tilt_angle = rep_tilt_angles(i);
    
    B(1,i) = sin(arm_angles(i))*sin(tilt_angle);
    B(2,i) = -cos(arm_angles(i))*sin(tilt_angle);
    B(3,i) = cos(tilt_angle);
    B(4,i) = -(rotor_moment_constant*spin(i)*sin(tilt_angle) - cos(tilt_angle)*arm_length)*sin(arm_angles(i));
    B(5,i) =  (rotor_moment_constant*spin(i)*sin(tilt_angle) - cos(tilt_angle)*arm_length)*cos(arm_angles(i));
    B(6,i) = -(rotor_moment_constant*spin(i)*cos(tilt_angle) + sin(tilt_angle)*arm_length);
end

B = B*rotor_force_constant;

== matlab function omav_LBF_bisection_combined/Motors and Servos/MATLAB Function1 ==
  data: tilt_angles input; B output
function B = get_B(tilt_angles)
%tilt_angles [6x1]
%[F, tau] = B * [omega²]

params = parameters();

rotor_force_constant = params.rotor_force_constant;
rotor_moment_constant = params.rotor_moment_constant;
arm_length = params.arm_length;

arm_angles = params.arm_angles;
spin = params.spin;

B = zeros(6,12);


j = 0;

%repeat every tilt angle
rep_tilt_angles = repelem(tilt_angles,2);
%iterating through every rotor
%refactored to z-upwards
for i = 1:12
  
    tilt_angle = rep_tilt_angles(i);
    
    B(1,i) = sin(arm_angles(i))*sin(tilt_angle);
    B(2,i) = -cos(arm_angles(i))*sin(tilt_angle);
    B(3,i) = cos(tilt_angle);
    B(4,i) = -(rotor_moment_constant*spin(i)*sin(tilt_angle) - cos(tilt_angle)*arm_length)*sin(arm_angles(i));
    B(5,i) =  (rotor_moment_constant*spin(i)*sin(tilt_angle) - cos(tilt_angle)*arm_length)*cos(arm_angles(i));
    B(6,i) = -(rotor_moment_constant*spin(i)*cos(tilt_angle) + sin(tilt_angle)*arm_length);
end

B = B*rotor_force_constant;

== matlab function omav_LBF_bisection_combined/new_control/Position Control/desired force/MATLAB Function1 ==
  data: tilt_angles input; B output
function B = get_B(tilt_angles)
%tilt_angles [6x1]
%[F, tau] = B * [omega²]

params = parameters();

rotor_force_constant = params.rotor_force_constant;
rotor_moment_constant = params.rotor_moment_constant;
arm_length = params.arm_length;

arm_angles = params.arm_angles;
spin = params.spin;

B = zeros(6,12);


j = 0;

%repeat every tilt angle
rep_tilt_angles = repelem(tilt_angles,2);
%iterating through every rotor
%refactored to z-upwards
for i = 1:12
  
    tilt_angle = rep_tilt_angles(i);
    
    B(1,i) = sin(arm_angles(i))*sin(tilt_angle);
    B(2,i) = -cos(arm_angles(i))*sin(tilt_angle);
    B(3,i) = cos(tilt_angle);
    B(4,i) = -(rotor_moment_constant*spin(i)*sin(tilt_angle) - cos(tilt_angle)*arm_length)*sin(arm_angles(i));
    B(5,i) =  (rotor_moment_constant*spin(i)*sin(tilt_angle) - cos(tilt_angle)*arm_length)*cos(arm_angles(i));
    B(6,i) = -(rotor_moment_constant*spin(i)*cos(tilt_angle) + sin(tilt_angle)*arm_length);
end

B = B*rotor_force_constant;

== matlab function omav_LBF_bisection_combined/EOM/MATLAB Function1 ==
  data: R_ input; R output
function R = normalize_rotmat(R_)
%normalize R every step to guarantee that R is orthogonal matrix (valid
%rotation)
[U,~,V] = svd(R_);
R = U*V';

== matlab function omav_LBF_bisection_combined/EOM/MATLAB Function ==
  data: x input; x_hat output
function x_hat = hat_map(x)
x_hat = [0 -x(3) x(2); x(3) 0 -x(1); -x(2) x(1) 0];

== matlab function omav_LBF_bisection_combined/new_control/B_wrench_mapper/MATLAB Function2 ==
  data: B input; omega_sq output; wrench_b input
function omega_sq = get_omegasq(B,wrench_b)
%GET_OMEGASQ Summary of this function goes here
%   Detailed explanation goes here

params = parameters();
omega_sq = pinv(B)*wrench_b;

for i = 1:12
    if omega_sq(i) < 0
        omega_sq(i) = 0;
    end
    
    if omega_sq(i) > (params.rotor_max)^2
        omega_sq(i) = (params.rotor_max)^2;
    end
end

end

== matlab function omav_LBF_bisection_combined/old_control/A_allocation/MATLAB Function3 ==
  data: A output
function A = get_A()
%[F, tau] = A * [sin(alpha)*omega², cos(alpha)*omega²]

params = parameters();

rotor_force_constant = params.rotor_force_constant;
rotor_moment_constant = params.rotor_moment_constant;
arm_length = params.arm_length;

arm_angles = params.arm_angles;
spin = params.spin;

%implementing pre-calculated matrix
%zero entries are commented out
A = zeros(6,24);

%iterating through every rotor
%refactored to z-up coordinate system
for i = 1:12
    A(1,2*i-1) = sin(arm_angles(i));
    %A(1,2*i) = 0;
    
    A(2,2*i-1) = -cos(arm_angles(i));
    %A(2,2*i) = 0;
    
    %A(3,2*i-1) = 0;
    A(3,2*i) = 1;
    
    A(4,2*i-1) = -rotor_moment_constant*spin(i)*sin(arm_angles(i));
    A(4,2*i) = sin(arm_angles(i))*arm_length;
    
    A(5,2*i-1) = rotor_moment_constant*spin(i)*cos(arm_angles(i));
    A(5,2*i) = -cos(arm_angles(i))*arm_length;
    
    A(6,2*i-1) = -arm_length;
    A(6,2*i) = -rotor_moment_constant*spin(i);
end

%multiplying with rotor force constant
A = A*rotor_force_constant;

== matlab function omav_LBF_bisection_combined/old_control/A_allocation/MATLAB Function4 ==
  data: X input; alphas output; omegas_sq output
function [alphas, omegas_sq] = get_projections(X)
%GET_PROJECTIONS Summary of this function goes here
%   Detailed explanation goes here


%get the angles
alphas = zeros(6,1);
for i = 1:6
    %get to entry which corresponds to arm
    j = 4*i - 3;
    alphas(i) = atan2(X(j)+X(j+2),X(j+1)+X(j+3));
end

omegas_sq = zeros(12,1);
for i = 1:6
    %get to entry which corresponds to arm
    j = 4*i - 3;
    
    omegas_sq(2*i-1) = X(j)*sin(alphas(i)) + X(j+1)*cos(alphas(i));
    omegas_sq(2*i)   = X(j+2)*sin(alphas(i)) + X(j+3)*cos(alphas(i));
end

%set to zero if smaller than zero
for i = 1:12
    if omegas_sq(i) < 0
        omegas_sq(i) = 0;
    end
end

== matlab function omav_LBF_bisection_combined/old_control/A_allocation/MATLAB Function5 ==
  data: A input; X output; wrench_b input
function X = get_X(A,wrench_b)
%GET_X Summary of this function goes here
%   Detailed explanation goes here
wrench_b = wrench_b(:);

X = pinv(A)*wrench_b;
end

== matlab function omav_LBF_bisection_combined/new_control/B_wrench_mapper/MATLAB Function6 ==
  data: tilt_angles input; B output
function B = get_B(tilt_angles)
%tilt_angles [6x1]
%[F, tau] = B * [omega²]

params = parameters();

rotor_force_constant = params.rotor_force_constant;
rotor_moment_constant = params.rotor_moment_constant;
arm_length = params.arm_length;

arm_angles = params.arm_angles;
spin = params.spin;

B = zeros(6,12);


j = 0;

%repeat every tilt angle
rep_tilt_angles = repelem(tilt_angles,2);
%iterating through every rotor
%refactored to z-upwards
for i = 1:12
  
    tilt_angle = rep_tilt_angles(i);
    
    B(1,i) = sin(arm_angles(i))*sin(tilt_angle);
    B(2,i) = -cos(arm_angles(i))*sin(tilt_angle);
    B(3,i) = cos(tilt_angle);
    B(4,i) = -(rotor_moment_constant*spin(i)*sin(tilt_angle) - cos(tilt_angle)*arm_length)*sin(arm_angles(i));
    B(5,i) =  (rotor_moment_constant*spin(i)*sin(tilt_angle) - cos(tilt_angle)*arm_length)*cos(arm_angles(i));
    B(6,i) = -(rotor_moment_constant*spin(i)*cos(tilt_angle) + sin(tilt_angle)*arm_length);
end

B = B*rotor_force_constant;

== matlab function omav_LBF_bisection_combined/References/MATLAB Function7 ==
  data: yaw_pitch_roll input; rotm output
function rotm = fcn(yaw_pitch_roll)
yaw_pitch_roll = yaw_pitch_roll(:)';
rotm = eul2rotm(yaw_pitch_roll);

== matlab function omav_LBF_bisection_combined/new_control/Attitude Control/attitude_error_calculation/MATLAB Function8 ==
  data: mat input; vec output
function vec = vee_map(mat)

vec = [-mat(2,3); mat(1,3); -mat(1,2)];

== matlab function omav_LBF_bisection_combined/new_control/Position Control/desired force/MATLAB Function ==
  data: B input; I_f_r input; B_f_c output; R input; lambda output
function [B_f_c,lambda] = get_reference_force_rotated(B,I_f_r, R)

params = parameters();

% get force vector in body frame
B_f_r = R'*I_f_r;

% sum columns to get main force direction
B_sum = sum(B(1:3,:),2);

% normalize to get unit vector
e_alpha = B_sum / norm(B_sum);

% get rotation matrix which to frame with e_alpha as 3rd axis
u = [0 0 1]';
v = e_alpha;

chi = 2*atan2(norm(norm(v)*u-norm(u)*v),norm(norm(v)*u+norm(u)*v));
n = cross(u,v);
axang = [n' chi];

if chi < 0.0001
    R_alpha = eye(3);
else
    R_alpha = axang2rotm(axang);
end

% get angle between e_alpha and B_f_r
u = e_alpha;
v = B_f_r;

lambda_r = 2*atan2(norm(norm(v)*u-norm(u)*v),norm(norm(v)*u+norm(u)*v));
n = cross(u,v);

% bisection search
B_pinv = pinv(B);

% parameter import
omega_sq_max = (params.f_omega_max)^2;
omega_sq_min = (params.f_omega_min)^2;
tol = params.f_tol;
delta_tol = params.f_delta_tol;
max_iter = params.f_max_iter;

lambda_min = 0;
lambda = lambda_min;

k=0;
delta = inf;

%allocate force vector
B_f_c = zeros(3,1);
while delta > delta_tol && k < max_iter 
    
    axang = [n' lambda];
    R_s = axang2rotm(axang);
    B_R_s = R_alpha*R_s;
    
    B_f_c = B_R_s*B_f_r;
    
    omega_sq = B_pinv * [R_s'*B_f_r;zeros(3,1)];
    
    %limit to positive values
    omega_sq = max(0,omega_sq);
    
    %limit to max rotor speed
    omega_sq = min(omega_sq_max,omega_sq);
    
    e_f = norm(B*omega_sq - [R_s'*B_f_r;zeros(3,1)]);
    
    if e_f < tol && max(omega_sq) < omega_sq_max && min(omega_sq) > omega_sq_min
        delta = 0.5*(lambda-lambda_min);
        lambda = lambda - delta;
    else
        lambda_min = lambda;
        delta = 0.5*(lambda_r - lambda);
        lambda = lambda + delta;
    end
    
    %increment loop counter
    k=k+1;
end

end

== matlab function omav_LBF_bisection_combined/old_control/A_allocation_wrench/MATLAB Function3 ==
  data: mat input; vec output
function vec = vee_map(mat)

vec = [-mat(2,3); mat(1,3); -mat(1,2)];

== matlab function omav_LBF_bisection_combined/new_control/Position Control/desired orientation/MATLAB Function1 ==
  data: B input; R_r input; R_s output; I_f_r input; lambda output
function [R_s,lambda] = get_search_rotmat(B,R_r,I_f_r)
params = parameters();

% get force vector in reference frame
r_f_r = R_r'*I_f_r;

% sum columns to get main force direction
B_sum = sum(B(1:3,:),2);

% normalize to get unit vector
e_alpha = B_sum / norm(B_sum);

% get rotation matrix which to frame with e_alpha as 3rd axis
u = [0 0 1]';
v = e_alpha;

chi = 2*atan2(norm(norm(v)*u-norm(u)*v),norm(norm(v)*u+norm(u)*v));
n = cross(u,v);
axang = [n' chi];

if chi < 0.0001
    R_alpha = eye(3);
else
    R_alpha = axang2rotm(axang);
end

% get angle between e_alpha and r_f_r
u = e_alpha;
v = r_f_r;

lambda_r = 2*atan2(norm(norm(v)*u-norm(u)*v),norm(norm(v)*u+norm(u)*v));
n = cross(u,v);

% bisection search
B_pinv = pinv(B);

% parameter import
omega_sq_max = (params.R_s_omega_max)^2;
omega_sq_min = (params.R_s_omega_min)^2;
tol = params.R_s_tol;
delta_tol = params.R_s_delta_tol;
max_iter = params.R_s_max_iter;

% lambda initialization
lambda_min = 0;
lambda = lambda_min;

k=0;
delta = inf;

%allocate Rotation Matrix
R_s = eye(3);
while delta > delta_tol && k < max_iter 
    
    axang = [n' lambda];
    R_s = axang2rotm(axang);
    
    omega_sq = B_pinv * [R_s'*r_f_r;zeros(3,1)];
    
    %limit to positive values
    omega_sq = max(0,omega_sq);
    
    %limit to max rotor speed
    omega_sq = min(omega_sq_max,omega_sq);
    
    e_f = norm(B*omega_sq - [R_s'*r_f_r;zeros(3,1)]);
    
    if e_f < tol && max(omega_sq) < omega_sq_max && min(omega_sq) > omega_sq_min
        delta = 0.5*(lambda-lambda_min);
        lambda = lambda - delta;
    else
        lambda_min = lambda;
        delta = 0.5*(lambda_r - lambda);
        lambda = lambda + delta;
    end
    
    %increment loop counter
    k=k+1;  
end

end
